simulink model "finalmodel15_10_org"  (Simulink 10.0)
settings: Solver=ode45  StartTime=0.0  StopTime=5  RelTol=1e-3  EnableMultiTasking=on
undefined symbols (not defined in the file): BCM1, Cadmium, Hydride, Metal, Nickel
libraries: powerlib x49, electricdrivelib x38, powerlib_meascontrol x5, powerlib_extras x3, simulink x2, fuzblock x1, fl_lib x1, re_lib x1
(part 2 of 2)

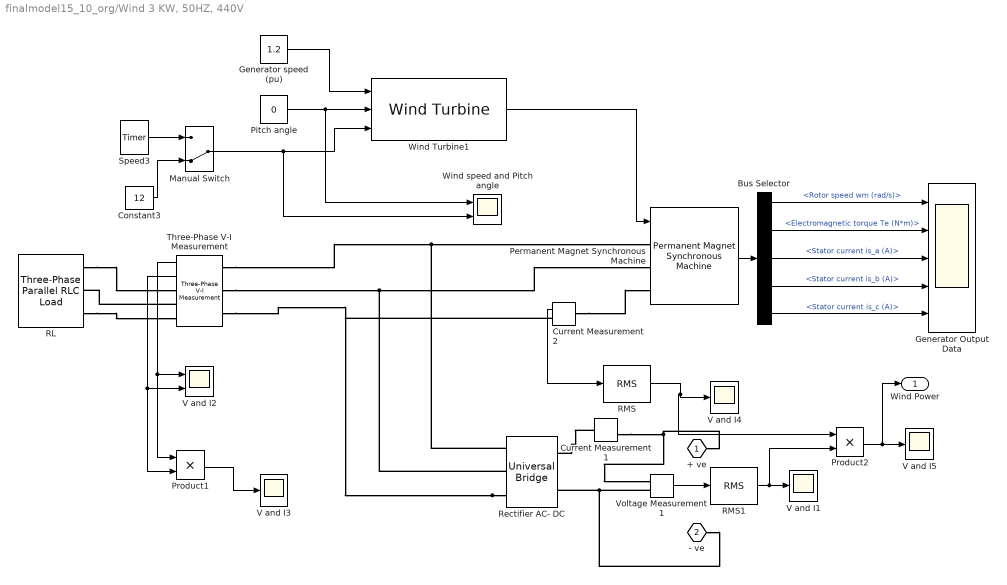
== system finalmodel15_10_org/Wind 3 KW, 50HZ, 440V ==
  Bus Selector : BusSelector  OutputSignals=Rotor speed wm (rad/s),Electromagnetic torque Te (N*m),Stator current is_a (A),Stator current is_b (A),Stator current is_c (A)
  Constant3 : Constant  Value=12
  Current Measurement1 : powerlib/Measurements/Current Measurement  PhasorSimulation=off  OutputType=Complex  PSBequivalent=0
      settings: SourceProductName=Simscape Electrical
  Current Measurement2 : powerlib/Measurements/Current Measurement  PhasorSimulation=off  OutputType=Complex  PSBequivalent=0
      settings: SourceProductName=Simscape Electrical
  Generator Output Data : Scope  NumInputPorts=5
  Generator speed (pu) : Constant  Value=1.2
  Manual Switch : ManualSwitch  CurrentSetting=0
  Permanent Magnet Synchronous Machine : powerlib/Machines/Permanent Magnet Synchronous Machine  NbPhases=3  FluxDistribution=Sinusoidal  RotorType=Round  MechanicalLoad=Torque Tm  PresetModel="05:  8 Nm 300 Vdc 2000 RPM - 10 Nm"  ShowDetailedParameters=on  MeasurementBus=off  Resistance=0.9585  Inductance=8.5e-3  dqInductances=[8.5e-3,8.5e-3]  La=0.00525  MachineConstant=Flux linkage established by magnets (V.s)  Flux=0.1827  VoltageCst=132.5525  TorqueCst=1.0962  Flat=120  Mechanical=[0.0006329 0.0003035 4 0]  PolePairs=4  InitialConditions=[0,0, 0,0]  InitialConditions5ph=[0 0 0 0 0 0]  RefAngle=90 degrees behind phase A axis (modified Park)  IterativeDiscreteModel=Trapezoidal non iterative  TsBlock=-1  TsPowergui=0
  Pitch angle : Constant  Value=0
  Product1 : Product
  Product2 : Product
  "RL " : powerlib/Elements/Three-Phase Parallel RLC Load  LConnTagsString=A|B|C  Configuration=Y (grounded)  NominalVoltage=400  Vabc=[1e3 1e3 1e3]  Vabcp=[1e3 1e3 1e3]  NominalFrequency=50  UnbalancedPower=off  ActivePower=5  InductivePower=1  CapacitivePower=0  Pabc=[10e3 9e3 11e3]  QLabc=[100 90 110]  QCabc=[100 90 110]  Pabcp=[10e3 9e3 11e3]  QLabcp=[100 90 110]  QCabcp=[100 90 110]  Measurements=None  LoadType=constant Z
      settings: SourceProductName=Simscape Electrical
  RMS : powerlib_meascontrol/Measurements/RMS  TrueRMS=on  Freq=50  RMSInit=1  Ts=0
      settings: SourceProductName=Simscape Electrical
  RMS1 : powerlib_meascontrol/Measurements/RMS  TrueRMS=on  Freq=50  RMSInit=1  Ts=0
      settings: SourceProductName=Simscape Electrical
  Rectifier AC- DC : powerlib/Power Electronics/Universal Bridge  Arms=3  SnubberResistance=1e5  SnubberCapacitance=inf  Device=Diodes  Ron=1e-3  Lon=0  ForwardVoltages="[  0  0  ]"  ForwardVoltage=0  GTOparameters=[ 10e-6 , 20e-6 ]  IGBTparameters=[ 1e-6 , 2e-6 ]  Measurements=None  Measurements_2=None  converterType=Rectifier
      settings: SourceProductName=Simscape Electrical
  Speed3 : powerlib_extras/Control  Blocks/Timer  t=[0 1 2]  e=[12 8 12]
      settings: SourceProductName=Simscape Electrical  SourceProductBaseCode=PS
  Three-Phase V-I Measurement : powerlib/Measurements/Three-Phase V-I Measurement  VoltageMeasurement=phase-to-ground  SetLabelV=off  LabelV=Vabc  Vpu=off  VpuLL=off  CurrentMeasurement=yes  SetLabelI=off  LabelI=Iabc  Ipu=off  Pbase=100e6  Vbase=500e3  OutputType=Complex  PhasorSimulation=off  PSBequivalent=0
      settings: SourceProductName=Simscape Electrical
  V and I{1,3..5} (4 alike) : Scope
  V and I2 : Scope  NumInputPorts=2
  Voltage Measurement1 : powerlib/Measurements/Voltage Measurement  PhasorSimulation=off  OutputType=Complex  PSBequivalent=0
      settings: SourceProductName=Simscape Electrical
  Wind Turbine1 : re_lib/Wind Generation/Wind Turbine  Pnom=5000  Pelec_base=190/.9  wind_base=12  P_wind_base=0.73  speed_nom=1.2  pitch_angle=0  c1_c6="[0.51763          116          0.4            5           21     0.006795]"  cp_nom=0.48  lambda_nom=8.1
      settings: SourceProductName=Simscape Electrical  SourceProductBaseCode=PS
  Wind speed and Pitch angle : Scope  NumInputPorts=2
  + ve : PMIOPort  Side=Right
  - ve : PMIOPort  Port=2  Side=Right
  Wind Power : Outport
  wires:
  Wind Turbine1/1 -> Permanent Magnet Synchronous Machine/1
  Pitch angle/1 -> Wind Turbine1/2, Wind speed and Pitch angle/1
  Generator speed (pu)/1 -> Wind Turbine1/1
  Permanent Magnet Synchronous Machine/1 -> Bus Selector/1
  Bus Selector/1 -> Generator Output Data/1  "<Rotor speed wm (rad/s)>"
  Bus Selector/2 -> Generator Output Data/2  "<Electromagnetic torque Te (N*m)>"
  Bus Selector/3 -> Generator Output Data/3  "<Stator current is_a (A)>"
  Bus Selector/4 -> Generator Output Data/4  "<Stator current is_b (A)>"
  Bus Selector/5 -> Generator Output Data/5  "<Stator current is_c (A)>"
  Speed3/1 -> Manual Switch/1
  Constant3/1 -> Manual Switch/2
  Manual Switch/1 -> Wind Turbine1/3, Wind speed and Pitch angle/2
  Three-Phase V-I Measurement/1 -> Product1/1, V and I2/1
  Three-Phase V-I Measurement/2 -> Product1/2, V and I2/2
  Product1/1 -> V and I3/1
  Current Measurement2/1 -> RMS/1
  Voltage Measurement1/1 -> RMS1/1
  RMS1/1 -> Product2/2, V and I1/1
  RMS/1 -> Product2/1, V and I4/1
  Product2/1 -> Wind Power/1, V and I5/1
  connections:
  Three-Phase V-I Measurement/LConn2 -- Rectifier AC- DC/LConn2 -- Permanent Magnet Synchronous Machine/LConn2
  Rectifier AC- DC/LConn3 -- Three-Phase V-I Measurement/LConn3 -- Current Measurement2/RConn1
  Three-Phase V-I Measurement/LConn1 -- Rectifier AC- DC/LConn1 -- Permanent Magnet Synchronous Machine/LConn1
  Voltage Measurement1/LConn2 -- - ve/RConn1 -- Rectifier AC- DC/RConn2
  Current Measurement1/RConn1 -- Voltage Measurement1/LConn1 -- + ve/RConn1
  Current Measurement1/LConn1 -- Rectifier AC- DC/RConn1
  Current Measurement2/LConn1 -- Permanent Magnet Synchronous Machine/LConn3
  "RL "/LConn1 -- Three-Phase V-I Measurement/RConn1
  Three-Phase V-I Measurement/RConn2 -- "RL "/LConn2
  "RL "/LConn3 -- Three-Phase V-I Measurement/RConn3

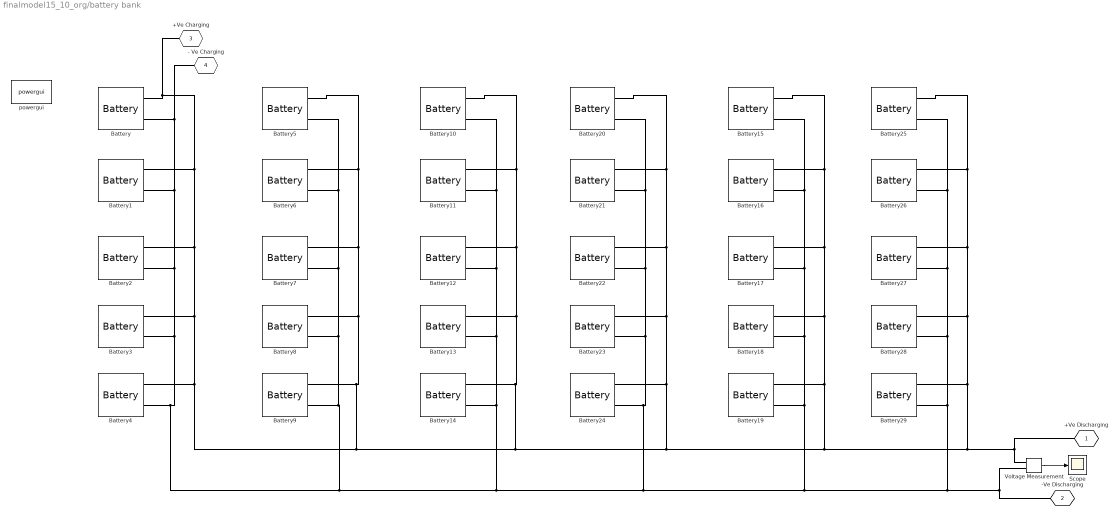
== system finalmodel15_10_org/battery bank  ==
  Battery{,5,10,15,20,25} (6 alike) : electricdrivelib/Extra Sources/Battery  BatType=Nickel-Cadmium  ShowTempParam=off  ThermalPreset=no  ShowAgeParam=off  NomV=43  NomQ=100  SOC=100  Batt_Tr=30  PresetModel=off  MaxQ=64  MinV=32.25  FullV=230  Dis_rate=20  R=0.0043  Normal_OP=96.1364  expZone="[45.8835      27.9545]"  current=[6.5 13 32.5]  Units=Time  Tci=20  NomT=20  T2=-30  MaxQ2=4.8  FullV2=7.1  Normal_OP2=5.655  expZone2="[6.58           1]"  Rca=0.6  ti=2000  Dp=0  Neq0=0  Tsim=1e6  Ta1=25  Qeol=5.4*0.9  Reol=0.013333*1.2  Char_age=[2.3478, 3]  Dis_age=[2.3478, 10]  N1=1500  N2=10500  N3=1000  N4=1400  Ta2=45  N5=950
      settings: SourceProductName=Simscape Electrical
  Battery{1..4,6..9,11..14,16..19,21..24,26..29} (24 alike) : electricdrivelib/Extra Sources/Battery  BatType=Nickel-Metal-Hydride  ShowTempParam=off  ThermalPreset=no  ShowAgeParam=off  NomV=43  NomQ=100  SOC=100  Batt_Tr=30  PresetModel=off  MaxQ=64  MinV=32.25  FullV=230  Dis_rate=20  R=0.0043  Normal_OP=96.1538  expZone="[46.6441           20]"  current=[6.5 13 32.5]  Units=Time  Tci=20  NomT=20  T2=-30  MaxQ2=4.8  FullV2=7.1  Normal_OP2=5.655  expZone2="[6.58           1]"  Rca=0.6  ti=2000  Dp=0  Neq0=0  Tsim=1e6  Ta1=25  Qeol=5.4*0.9  Reol=0.013333*1.2  Char_age=[2.3478, 3]  Dis_age=[2.3478, 10]  N1=1500  N2=10500  N3=1000  N4=1400  Ta2=45  N5=950
      settings: SourceProductName=Simscape Electrical
  Scope : Scope
  Voltage Measurement : powerlib/Measurements/Voltage Measurement  PhasorSimulation=off  OutputType=Complex  PSBequivalent=0
      settings: SourceProductName=Simscape Electrical
  powergui : powerlib/powergui  Priority=1  SimulationMode=Discrete  SampleTime=50e-6  frequency=60  Iterations=50  frequencyindice=0  Pbase=100e6  ErrMax=1e-4  UnitsV=kV  UnitsW=MW  buscounter=0  FunctionMessages=off  echomessages=off  EnableUseOfTLC=off  CurrentSourceSwitches=off  DisableSnubberDevices=off  DisableRonSwitches=off  DisableVfSwitches=off  DisplayEquations=off  AutomaticDiscreteSolvers=off  SolverType=Tustin  Interpol=off  ExternalGateDelay=off  methode=off  Ts=100  x0status=blocks  SPID=off  SwTol=0  HookPort=off  NonlinearTolerance=1e-4  nMaxIteration=100  ContinueOnMaxIteration=off  RestoreLinks=warning  ResistiveCurrentMeasurement=off  Frange=[0:2:500]  Ylog=off  Xlog=on  ShowGrid=off  save=off  variable=ZData  structure=0  ZoomFFT=off  StartTime=0.0  cycles=1  DisplayStyle=1  fundamental=60  FreqAxis=off  MaxFrequency=1000  frequencyindicesteady=1  RmsSteady=1  display=off
      settings: SourceProductName=Simscape Electrical
  +Ve Discharging : PMIOPort  Side=Right
  "-Ve Discharging " : PMIOPort  Port=2  Side=Right
  +Ve Charging : PMIOPort  Port=3  Side=Left
  - Ve Charging : PMIOPort  Port=4  Side=Left
  wires:
  Voltage Measurement/1 -> Scope/1
  connections:
  Battery25/LConn1 -- Voltage Measurement/LConn1 -- +Ve Discharging/RConn1 -- Battery19/LConn1 -- Battery15/LConn1 -- Battery16/LConn1 -- Battery17/LConn1 -- Battery18/LConn1 -- Battery23/LConn1 -- Battery22/LConn1 -- Battery21/LConn1 -- Battery20/LConn1 -- Battery24/LConn1 -- Battery13/LConn1 -- Battery12/LConn1 -- Battery11/LConn1 -- Battery10/LConn1 -- Battery14/LConn1 -- Battery8/LConn1 -- Battery7/LConn1 -- Battery5/LConn1 -- Battery6/LConn1 -- Battery9/LConn1 -- Battery/LConn1 -- +Ve Charging/RConn1 -- Battery1/LConn1 -- Battery2/LConn1 -- Battery3/LConn1 -- Battery4/LConn1 -- Battery29/LConn1 -- Battery28/LConn1 -- Battery27/LConn1 -- Battery26/LConn1
  Battery9/LConn2 -- Battery13/LConn2 -- Battery12/LConn2 -- Battery11/LConn2 -- Battery10/LConn2 -- Battery14/LConn2 -- Battery23/LConn2 -- Battery22/LConn2 -- Battery21/LConn2 -- Battery20/LConn2 -- Battery24/LConn2 -- Battery19/LConn2 -- Battery15/LConn2 -- Battery16/LConn2 -- Battery17/LConn2 -- Battery18/LConn2 -- Battery28/LConn2 -- Battery27/LConn2 -- Battery26/LConn2 -- Battery25/LConn2 -- Battery29/LConn2 -- "-Ve Discharging "/RConn1 -- Voltage Measurement/LConn2 -- - Ve Charging/RConn1 -- Battery/LConn2 -- Battery1/LConn2 -- Battery2/LConn2 -- Battery3/LConn2 -- Battery4/LConn2 -- Battery8/LConn2 -- Battery7/LConn2 -- Battery5/LConn2 -- Battery6/LConn2

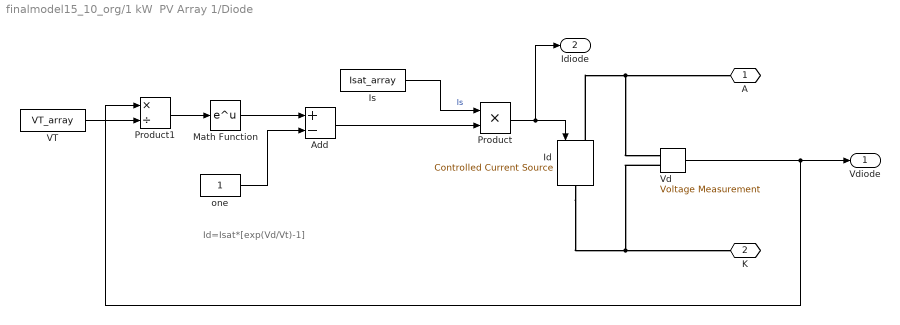
== system finalmodel15_10_org/1 kW  PV Array 1/Diode ==
  note: Id=Isat*[exp(Vd/Vt)-1]
  Add : Sum  Inputs=+-
  Id : powerlib/Electrical Sources/Controlled Current Source  Initialize=on  Source_Type=AC  Amplitude=0  Phase=0  Frequency=0  Measurements=None
      settings: SourceProductName=Simscape Electrical
  Is : Constant  Value=Isat_array
  Math Function : Math  SaturateOnIntegerOverflow=on
  Product : Product  RndMeth=Zero
  Product1 : Product  Inputs=*/  RndMeth=Zero
  VT : Constant  Value=VT_array
  Vd : powerlib/Measurements/Voltage Measurement  PhasorSimulation=off  OutputType=Complex  PSBequivalent=0
      settings: SourceProductName=Simscape Electrical
  one : Constant
  A : PMIOPort  Side=Left
  K : PMIOPort  Port=2  Side=Right
  Vdiode : Outport
  Idiode : Outport  Port=2
  wires:
  VT/1 -> Product1/2
  Add/1 -> Product/2
  one/1 -> Add/2
  Product1/1 -> Math Function/1
  Is/1 -> Product/1  "Is"
  Vd/1 -> Vdiode/1, Product1/1
  Product/1 -> Id/1, Idiode/1
  Math Function/1 -> Add/1
  connections:
  Id/LConn1 -- A/RConn1 -- Vd/LConn1
  Vd/LConn2 -- K/RConn1 -- Id/RConn1
